simulink model "chap4_3sim"  (Simulink 7.0)
settings: Solver=ode45  StartTime=0.0  StopTime=20  RelTol=1e-5
settings Model: Creator=hp  LastModifiedBy=eleliuj  ExtModeTrigMode=oneshot  ExtModeArmWhenConnect=off
settings DataIOCC: LimitDataPoints=off  SignalLoggingName=sigsOut
settings OptimizationCC: BooleanDataType=off
settings DebuggingCC: SaveWithParameterizedLinksMsg=none  SignalResolutionControl=TryResolveAllWithWarning  SolverPrmCheckMsg=none  MultiTaskDSMMsg=warning  MultiTaskCondExecSysMsg=none
settings HardwareCC: TargetUnknown=on
settings RTWCC: IncludeERTFirstTime=on
settings GRTTargetCC: TargetFcnLib=ansi_tfl_tmw.mat

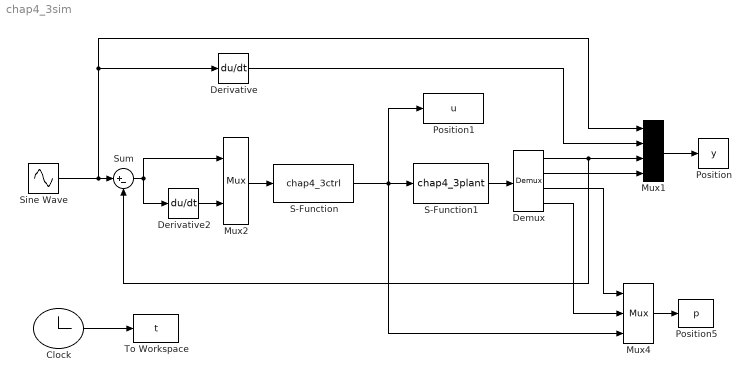
== system chap4_3sim ==
  Clock : Clock
      settings: Decimation=10
  Demux : Demux
  Derivative : Derivative
  Derivative2 : Derivative
  Mux1 : Mux
  Mux2 : Mux  Inputs=2
  Mux4 : Mux  Inputs=3
  Position : ToWorkspace  VariableName=y  SampleTime=-1  SaveFormat=Array
  Position1 : ToWorkspace  VariableName=u  SampleTime=-1  SaveFormat=Array
  Position5 : ToWorkspace  VariableName=p  SampleTime=-1  SaveFormat=Array
  S-Function : S-Function  FunctionName=chap4_3ctrl
  S-Function1 : S-Function  FunctionName=chap4_3plant
  Sine Wave : Sin  SampleTime=0
  Sum : Sum  Inputs=|+-  OutDataType=sfix(16)  OutScaling=2^0  SaturateOnIntegerOverflow=on
  To Workspace : ToWorkspace  VariableName=t  SampleTime=-1  SaveFormat=Array
  wires:
  Mux1/1 -> Position/1
  Demux/1 -> Sum/2, Mux1/3
  S-Function1/1 -> Demux/1
  Clock/1 -> To Workspace/1
  Mux4/1 -> Position5/1
  Sine Wave/1 -> Sum/1, Mux1/1, Derivative/1
  Mux2/1 -> S-Function/1
  Sum/1 -> Mux2/1, Derivative2/1
  Derivative2/1 -> Mux2/2
  Demux/3 -> Mux4/1
  S-Function/1 -> S-Function1/1, Position1/1, Mux4/3
  Demux/4 -> Mux4/2
  Demux/2 -> Mux1/4
  Derivative/1 -> Mux1/2
